simulink model "hybrid_lht_accumulator_backup"  (R2019b)
settings: Solver=FixedStepDiscrete  StartTime=0.0  StopTime=inf  FixedStep=1/bt.frequency  RelTol=1e-3
InitFcn:
  | ht_hybrid_setup;
StopFcn:
  | ht_hybrid_compare;
undefined symbols (not defined in the file or in its folder): bt, height, Ntheta, nTheta, width
libraries: hdlsllib x52, simulink x24, visionhdlutilities x2, dspsrcs4 x1, visionhdlio x1, lib_hybrid_ht_kernel x1, visionsources x1
(part 4 of 5)

== system hybrid_lht_accumulator_backup/Hybrid LHT2/Hybrid LHT Accumulator/Accumulator with Switches/Accumulator/Block RAM ==
  wr_data : Inport
  wr_addr : Inport  Port=2
  wr_en : Inport  Port=3
  rd_addr : Inport  Port=4
  Simple Dual Port RAM : Subsystem  VariantControl=9_bits
  Simple Dual Port RAM Generator : Subsystem  VariantControl=other_bits  mask{b=36, d=400, b_hidden=12, d_hidden=2204}
      mask prompts: b "Data width:"; d "Depth:"
      mask init:
      | if b == b_hidden && d == d_hidden
      |     return
      | end
      | 
      | % Xilinx RAM Initialisation
      | xl_config = [512, 72;
      |             1024, 36;
      |             2048, 18;
      |             4096, 9;
      |             8192, 4;
      |             16384, 2;
      |             32768, 1];
      | 
      | % Get length of Xilinx Configuration
      | sizeram = size(xl_config);
      |         
      | % Get the RAM Configuration based on the data width
      | for i = 1:sizeram(1)
      |     if b <= xl_config(i, 2)
      |         a = xl_config(i, :);
      |     end
      | end
      | 
      | % Get number of BRAM required (including half BRAM)
      | numbram = ceil((d/a(1))/0.5)*0.5;
      | fullbram = floor(numbram); % Integer
      | halfbram = (numbram-floor(numbram)) ~= 0; % Boolean
      | 
      | % Get all blocks and delete everything excepts ports
      | H = get(find_system(gcb, 'FindAll', 'on', 'type', 'block'));
      | todelete = setdiff(strcat(repmat({[gcb '/']}, numel(H.Blocks), 1),  H.Blocks),...
      |     strcat(repmat({[gcb '/']}, 5, 1),...
      |     {'wr_data'; 'wr_addr'; 'wr_en'; 'rd_addr'; 'rd_data'}));
      | delete_block(todelete);
      | 
      | % Delete lines
      | for i = 1:numel(H.Lines)
      |     delete_line(H.Lines(i).Handle)
      | end
      | 
      | % Generate full BRAMs
      | y = 0;
      | 
      | % If there is only one ram then the write enable should be directly
      | % connected to the first ram write enable. Else, the write address must be sliced
      | % and the upper bound (over a(2)) compared to zero. This will indicate if
      | % the first ram is the one to be written/read from.
      | 
      | % Common to both implementations
      | % Write Address Slice
      | add_block('hdlsllib/Logic and Bit Operations/Bit Slice',...
      |         [gcb, '/wr_address'], 'Position',...
      |         [160 130 250 170]);
      | % Set bitslice parameters
      | set_param([gcb, '/wr_address'],...
      |     'lidx', int2str(log2(a(1))-1));
      | set_param([gcb, '/wr_address'],...
      |     'ridx', int2str(0));
      | 
      | % Read Address Slice
      | add_block('hdlsllib/Logic and Bit Operations/Bit Slice',...
      |         [gcb, '/rd_address'], 'Position',...
      |         [160 330 250 370]);
      | % Set bitslice parameters
      | set_param([gcb, '/rd_address'],...
      |     'lidx', int2str(log2(a(1))-1));
      | set_param([gcb, '/rd_address'],...
      |     'ridx', int2str(0));
      | 
      | if ceil(numbram) == 1
      |     
      |     i = 1;
      |     
      |     % Add Simple RAM
      |     add_block('hdlsllib/HDL RAMs/Simple Dual Port RAM',...
      |         [gcb, '/simple_ram_', int2str(i-1)], 'Position',...
      |         [635 0+600*y 635+200 400+600*y]);
      | 
      |     % Set RAM parameters
      |     set_param([gcb, '/simple_ram_', int2str(i-1)],...
      |         'ram_size', int2str(log2(a(1))));
      | 
      |     % Connect "wr_data" to "simple_ram_i"
      |     add_line(gcb, ['wr_data/1'], ['simple_ram_', int2str(i-1), '/1'],...
      |         'autorouting', 'on');
      |     
      |     % Connect "wr_addr" to "wr_address"
      |     add_line(gcb, ['wr_addr/1'], ['wr_address/1'],...
      |         'autorouting', 'on');
      | 
      |     % Connect "wr_address" to "simple_ram_i"
      |     add_line(gcb, ['wr_address/1'], ['simple_ram_', int2str(i-1), '/2'],...
      |         'autorouting', 'on');
      | 
      |     % Connect "wr_en" to "simple_ram_i"
      |     add_line(gcb, ['wr_en/1'], ['simple_ram_', int2str(i-1), '/3'],...
      |         'autorouting', 'on');
      |     
      |     % Connect "rd_addr" to "rd_address"
      |     add_line(gcb, ['rd_addr/1'], ['rd_address/1'],...
      |         'autorouting', 'on');
      | 
      |     % Connect "rd_address" to "simple_ram_i"
      |     add_line(gcb, ['rd_address/1'], ['simple_ram_', int2str(i-1), '/4'],...
      |         'autorouting', 'on');
      | 
      |     % Connect "simple_ram_i" to "rd_data"
      |     add_line(gcb, ['simple_ram_', int2str(i-1), '/1'], ['rd_data/1'],...
      |         'autorouting', 'on');
      | 
      | else
      |     
      |     % Multiport Switch
      |     add_block('hdlsllib/Signal Routing/Multiport Switch',...
      |         [gcb, '/multiport_switch'], 'Position',...
      |         [1340 146 1405 250]);
      |     % Set multiport switch parameters
      |     set_param([gcb, '/multiport_switch'],...
      |         'Inputs', int2str(ceil(numbram)));
      |     set_param([gcb, '/multiport_switch'],...
      |         'DataPortOrder', 'Zero-based contiguous');
      | 
      |     % Add Constant Zero
      |     add_block('hdlsllib/Sources/Constant',...
      |         [gcb, '/zero'], 'Position',...
      |         [425 -65 455 -35]);
      |     set_param([gcb, '/zero'],...
      |         'Value', int2str(0));
      |     set_param([gcb, '/zero'],...
      |         'OutDataTypeStr', ['fixdt(0, ', int2str(ceil(numbram)), ', 0)']);
      | 
      |     % Add Vector Concatenate
      |     add_block('hdlsllib/Signal Routing/Vector Concatenate',...
      |         [gcb, '/vector_concatenate'], 'Position',...
      |         [1015, -113, 1025, 38]);
      |     set_param([gcb, '/vector_concatenate'],...
      |         'NumInputs', int2str(ceil(numbram)));
      | 
      |     % Add Bitwise-OR
      |     add_block('hdlsllib/Logic and Bit Operations/Bitwise Operator',...
      |         [gcb, '/bitwise_or'], 'Position',...
      |         [1165, -54, 1205, -16]);
      |     set_param([gcb, '/bitwise_or'],...
      |         'logicop', 'OR');
      |     set_param([gcb, '/bitwise_or'],...
      |         'UseBitMask', 0);
      |     set_param([gcb, '/bitwise_or'],...
      |         'NumInputPorts', int2str(1));
      | 
      |     % Add delay for bram access
      |     add_block('hdlsllib/Discrete/Delay',...
      |         [gcb, '/delay'], 'Position',...
      |         [1248, 60, 1282, 95]);
      |     set_param([gcb, '/delay'],...
      |         'DelayLength', int2str(1));
      |     
      |     % Add bitslice
      |     add_block('hdlsllib/Logic and Bit Operations/Bit Slice',...
      |         [gcb, '/wr_bitslice'], 'Position',...
      |         [-65 180 25 220]);
      | 
      |     % Set bitslice parameters
      |     set_param([gcb, '/wr_bitslice'],...
      |         'lidx', int2str(ceil(log2(d)-1)));
      |     set_param([gcb, '/wr_bitslice'],...
      |         'ridx', int2str(log2(a(1))));
      |     
      |     % Add bitslice
      |     add_block('hdlsllib/Logic and Bit Operations/Bit Slice',...
      |         [gcb, '/rd_bitslice'], 'Position',...
      |         [-65 280 25 320]);
      | 
      |     % Set bitslice parameters
      |     set_param([gcb, '/rd_bitslice'],...
      |         'lidx', int2str(ceil(log2(d)-1)));
      |     set_param([gcb, '/rd_bitslice'],...
      |         'ridx', int2str(log2(a(1))));
      |     
      |     for i = 1:ceil(numbram)
      |         
      |         %%%%% Begin Adding Blocks %%%%%
      |         % Add Simple RAM
      |         add_block('hdlsllib/HDL RAMs/Simple Dual Port RAM',...
      |             [gcb, '/simple_ram_', int2str(i-1)], 'Position',...
      |             [635 0+600*y 635+200 400+600*y]);
      | 
      |         % Set RAM parameters
      |         set_param([gcb, '/simple_ram_', int2str(i-1)],...
      |             'ram_size', int2str(log2(a(1))));
      | 
      |         % Add compare to constant
      |         add_block('hdlsllib/Logic and Bit Operations/Compare To Constant',...
      |             [gcb, '/wr_cmp2const_', int2str(i-1)], 'Position',...
      |             [190 225+y*600 220 255+y*600]); 
      | 
      |         % Set compare to zero parameters
      |         set_param([gcb, '/wr_cmp2const_', int2str(i-1)],...
      |             'relop', '==');
      | 
      |         % Set compare to zero parameters
      |         set_param([gcb, '/wr_cmp2const_', int2str(i-1)],...
      |             'const', int2str(i-1));
      |         
      |         % Add compare to constant
      |         add_block('hdlsllib/Logic and Bit Operations/Compare To Constant',...
      |             [gcb, '/rd_cmp2const_', int2str(i-1)], 'Position',...
      |             [190 445+y*600 220 475+y*600]); 
      | 
      |         % Set compare to zero parameters
      |         set_param([gcb, '/rd_cmp2const_', int2str(i-1)],...
      |             'relop', '==');
      | 
      |         % Set compare to zero parameters
      |         set_param([gcb, '/rd_cmp2const_', int2str(i-1)],...
      |             'const', int2str(i-1));
      | 
      |         % Add and logic
      |         add_block('hdlsllib/Logic and Bit Operations/Logical Operator',...
      |             [gcb, '/and_', int2str(i-1)], 'Position',...
      |             [420 231+600*y 455 264+600*y]);
      | 
      |         % Set and logic parameters
      |         set_param([gcb, '/and_', int2str(i-1)],...
      |             'Operator', 'AND');
      | 
      |         % Add Switch
      |         add_block('hdlsllib/Signal Routing/Switch',...
      |             [gcb, '/switch_', int2str(i-1)], 'Position',...
      |             [685 -113+600*y 785 -37+600*y]);
      | 
      |         % Set switch parameters
      |         set_param([gcb, '/switch_', int2str(i-1)],...
      |             'Threshold', int2str(1));
      | 
      |         % Add Constant
      |         add_block('hdlsllib/Sources/Constant',...
      |             [gcb, '/constant_', int2str(i-1)], 'Position',...
      |             [425 -115+600*y 455 -85+600*y]);
      | 
      |         % Set Constant parameters
      |         set_param([gcb, '/constant_', int2str(i-1)],...
      |             'Value', int2str(i-1));
      |         set_param([gcb, '/constant_', int2str(i-1)],...
      |             'OutDataTypeStr', ['fixdt(0, ', int2str(ceil(numbram)), ', 0)']);   
      | 
      |         %%%%% Begin Wire Connections %%%%%        
      |         % Connect "wr_data" to "simple_ram_i"
      |         add_line(gcb, 'wr_data/1', ['simple_ram_', int2str(i-1), '/1'],...
      |             'autorouting','on');
      | 
      |         % Connect "wr_address" to "simple_ram_i"
      |         add_line(gcb, 'wr_address/1', ['simple_ram_', int2str(i-1), '/2'],...
      |             'autorouting','on');
      | 
      |         % Connect "rd_address" to "simple_ram_i"
      |         add_line(gcb, 'rd_address/1', ['simple_ram_', int2str(i-1), '/4'],...
      |             'autorouting','on');
      | 
      |         % Connect "constant_i" to "switch_i"
      |         add_line(gcb, ['constant_', int2str(i-1), '/1'], ['switch_', int2str(i-1), '/1'],...
      |             'autorouting','on');
      | 
      |         % Connect "zero" to "switch_i"
      |         add_line(gcb, 'zero/1', ['switch_', int2str(i-1), '/3'],...
      |             'autorouting','on');
      | 
      |         % Connect "switch_i" to "vector_concatenate"
      |         add_line(gcb, ['switch_', int2str(i-1), '/1'], ['vector_concatenate/', int2str(i)],...
      |             'autorouting','on');
      | 
      |         % Connect "rd_address" to "simple_ram_i"
      |         add_line(gcb, ['simple_ram_', int2str(i-1), '/1'],['multiport_switch/', int2str(i+1)],...
      |             'autorouting','on');
      | 
      |         % Connect "bitslice_i" to "wr_cmp2const_i"
      |         add_line(gcb, ['wr_bitslice/1'], ['wr_cmp2const_', int2str(i-1), '/1'],...
      |             'autorouting','on');
      |         
      |         % Connect "bitslice_i" to "rd_cmp2const_i"
      |         add_line(gcb, ['rd_bitslice/1'], ['rd_cmp2const_', int2str(i-1), '/1'],...
      |             'autorouting','on');
      | 
      |         % Connect "wr_en" to "and_i"
      |         add_line(gcb, ['wr_en/1'], ['and_', int2str(i-1), '/2'],...
      |             'autorouting','on');
      | 
      |         % Connect "and_i" to "simple_ram_0"
      |         add_line(gcb, ['and_', int2str(i-1), '/1'], ['simple_ram_', int2str(i-1), '/3'],...
      |             'autorouting','on');
      | 
      |         % Connect "wr_cmp2const_i" to "and_i"
      |         add_line(gcb, ['wr_cmp2const_', int2str(i-1), '/1'], ['and_', int2str(i-1), '/1'],...
      |             'autorouting','on');
      | 
      |         % Connect "rd_cmp2const_i" to "switch_i"
      |         add_line(gcb, ['rd_cmp2const_', int2str(i-1), '/1'], ['switch_', int2str(i-1), '/2'],...
      |             'autorouting','on');
      |          
      |         % Update coordinates
      |         y = y + 1;
      |         
      |     end
      |     
      |     % Connect "rd_addr" to "bitslice_i"
      |     add_line(gcb, ['rd_addr/1'], ['rd_bitslice/1'],...
      |         'autorouting','on');
      |     
      |     % Connect "wr_addr" to "bitslice_i"
      |     add_line(gcb, ['wr_addr/1'], ['wr_bitslice/1'],...
      |         'autorouting','on');
      |     
      |     % Connect "wr_addr" to "wr_address"
      |     add_line(gcb, 'wr_addr/1', ['wr_address', '/1'],...
      |         'autorouting','on');
      | 
      |     % Connect "rd_addr" to "rd_address"
      |     add_line(gcb, 'rd_addr/1', ['rd_address', '/1'],...
      |         'autorouting','on');
      | 
      |     % Connect "vector_concatenate" to "bitwise_or"
      |     add_line(gcb, ['vector_concatenate/1'], ['bitwise_or/1'],...
      |         'autorouting','on');
      | 
      |     % Connect "bitwise_or" to "delay"
      |     add_line(gcb, ['bitwise_or/1'], ['delay/1'],...
      |         'autorouting','on');
      | 
      |     % Connect "delay" to "multiport_switch"
      |     add_line(gcb, ['delay/1'], ['multiport_switch/1'],...
      |         'autorouting','on');
      | 
      |     % Connect "multiport_switch" to "rd_data"
      |     add_line(gcb, ['multiport_switch/1'], ['rd_data/1'],...
      |         'autorouting','on');
      |     
      | end
      | 
      | % If there is a half bram we must change a few parameters. Firstly, delete
      | % the write and read address lines. Then add bitslice blocks to reduce the
      | % address space in half. Connect rd_addr and wr_addr to the corresponding ports
      | % on the bram. Finally, change the address depth.
      | if halfbram
      |     
      |     if ceil(numbram) > 1
      |         
      |         % Delete lines
      |         delete_line(gcb, ['wr_address/1'], ['simple_ram_', int2str(i-1), '/2'])
      |         delete_line(gcb, ['rd_address/1'], ['simple_ram_', int2str(i-1), '/4'])
      |         
      |         % Write Address half ram Slice
      |         add_block('hdlsllib/Logic and Bit Operations/Bit Slice',...
      |                 [gcb, '/wr_address_hr'], 'Position',...
      |                 [160 130+(y-1)*600 250 170+(y-1)*600]);
      |         % Set bitslice parameters
      |         set_param([gcb, '/wr_address_hr'],...
      |             'lidx', int2str(log2(a(1))-2));
      |         set_param([gcb, '/wr_address_hr'],...
      |             'ridx', int2str(0));
      | 
      |         % Read Address half ram Slice
      |         add_block('hdlsllib/Logic and Bit Operations/Bit Slice',...
      |                 [gcb, '/rd_address_hr'], 'Position',...
      |                 [160 330+(y-1)*600 250 370+(y-1)*600]);
      |         % Set bitslice parameters
      |         set_param([gcb, '/rd_address_hr'],...
      |             'lidx', int2str(log2(a(1))-2));
      |         set_param([gcb, '/rd_address_hr'],...
      |             'ridx', int2str(0));
      | 
      |         % Connect "wr_addr" to "wr_address_hr"
      |         add_line(gcb, 'wr_addr/1', ['wr_address_hr', '/1'],...
      |             'autorouting','on');
      | 
      |         % Connect "rd_addr" to "rd_address_hr"
      |         add_line(gcb, 'rd_addr/1', ['rd_address_hr', '/1'],...
      |             'autorouting','on');
      | 
      |         % Connect "wr_address_hr" to "simple_ram_i"
      |         add_line(gcb, ['wr_address_hr', '/1'], ['simple_ram_', int2str(i-1), '/2'],...
      |             'autorouting','on');
      | 
      |         % Connect "rd_address_hr" to "simple_ram_i"
      |         add_line(gcb, ['rd_address_hr', '/1'], ['simple_ram_', int2str(i-1), '/4'],...
      |             'autorouting','on');
      | 
      |     else
      |         % Set bitslice parameters
      |         set_param([gcb, '/wr_address'],...
      |             'lidx', int2str(log2(a(1))-2));
      |         set_param([gcb, '/wr_address'],...
      |             'ridx', int2str(0));
      |         % Set bitslice parameters
      |         set_param([gcb, '/rd_address'],...
      |             'lidx', int2str(log2(a(1))-2));
      |         set_param([gcb, '/rd_address'],...
      |             'ridx', int2str(0));
      |         
      |     end
      |     
      |     % Update the ram parameters (address bits)
      |     set_param([gcb, '/simple_ram_', int2str(i-1)],...
      |         'ram_size', int2str(log2(a(1)/2)));
      |     
      | end
      | 
      | b_hidden = b;
      | d_hiddne = d;
  rd_data : Outport

== system hybrid_lht_accumulator_backup/Hybrid LHT2/Hybrid LHT Accumulator2/Simple Hough Accumulator/Flag Generator/Flag Generator ==
  ReadOut : Inport
  Thresh : Inport  Port=2
  ZeroData : Inport  Port=3
  ReadValid : Inport  Port=4
  AND : Logic  IconShape=distinctive  AllPortsSameDT=off  OutDataTypeStr=boolean
  Bit Concat : hdlsllib/Logic and Bit Operations/Bit Concat  numInputs=2
      settings: SourceProductName=HDL Coder  SourceProductBaseCode=HD
  Relational Operator1 : RelationalOperator  OutDataTypeStr=boolean  RndMeth=Simplest
  ZeroDataFlagged : Outport  VectorParamsAs1DForOutWhenUnconnected=off
  wires:
  AND/1 -> Bit Concat/1
  ReadValid/1 -> AND/2
  Relational Operator1/1 -> AND/1
  ZeroData/1 -> Bit Concat/2
  Bit Concat/1 -> ZeroDataFlagged/1
  Thresh/1 -> Relational Operator1/2
  ReadOut/1 -> Relational Operator1/1

== system hybrid_lht_accumulator_backup/Hybrid LHT2/Hybrid LHT Accumulator2/Simple Hough Accumulator/Flag Generator/Passthrough ==
  ZeroData : Inport
  ZeroDataFlagged : Outport  VectorParamsAs1DForOutWhenUnconnected=off
  wires:
  ZeroData/1 -> ZeroDataFlagged/1

== system hybrid_lht_accumulator_backup/Hybrid LHT2/Hybrid LHT Accumulator2/Simple Hough Accumulator/Hough Accumulator/Simple Dual Port RAM Generator ==
  wr_data : Inport
  wr_addr : Inport  Port=2
  wr_en : Inport  Port=3
  rd_addr : Inport  Port=4
  rd_address : hdlsllib/Logic and Bit Operations/Bit Slice  lidx=8  ridx=0
      settings: SourceProductName=Simulink  SourceProductBaseCode=SL
  simple_ram_0 : hdlsllib/HDL RAMs/Simple Dual Port RAM  ram_size=9
      settings: SourceProductName=Simulink  SourceProductBaseCode=SL
  wr_address : hdlsllib/Logic and Bit Operations/Bit Slice  lidx=8  ridx=0
      settings: SourceProductName=Simulink  SourceProductBaseCode=SL
  rd_data : Outport
  wires:
  wr_data/1 -> simple_ram_0/1
  wr_addr/1 -> wr_address/1
  wr_address/1 -> simple_ram_0/2
  wr_en/1 -> simple_ram_0/3
  rd_addr/1 -> rd_address/1
  rd_address/1 -> simple_ram_0/4
  simple_ram_0/1 -> rd_data/1

== system hybrid_lht_accumulator_backup/Hybrid LHT2/Hybrid LHT Accumulator2/Simple Hough Accumulator/Keep Flag/Keep Flag ==
  FlagIn : Inport
  VoteIn : Inport  Port=2
  Bit Concat1 : hdlsllib/Logic and Bit Operations/Bit Concat  numInputs=2
      settings: SourceProductName=HDL Coder  SourceProductBaseCode=HD
  VoteFlagOut : Outport  VectorParamsAs1DForOutWhenUnconnected=off
  wires:
  VoteIn/1 -> Bit Concat1/2
  FlagIn/1 -> Bit Concat1/1
  Bit Concat1/1 -> VoteFlagOut/1

== system hybrid_lht_accumulator_backup/Hybrid LHT2/Hybrid LHT Accumulator2/Simple Hough Accumulator/Keep Flag/Passthrough ==
  FlagIn : Inport
  VoteIn : Inport  Port=2
  Terminator : Terminator
  VoteFlagOut : Outport  VectorParamsAs1DForOutWhenUnconnected=off
  wires:
  VoteIn/1 -> VoteFlagOut/1
  FlagIn/1 -> Terminator/1

== system hybrid_lht_accumulator_backup/Hybrid LHT2/Hybrid LHT Accumulator2/Simple Hough Accumulator/Separate Bits/Passthrough ==
  VoteFlagIn : Inport
  Constant : Constant  Value=0  OutDataTypeStr=boolean  SampleTime=-1
  FlagOut : Outport  VectorParamsAs1DForOutWhenUnconnected=off
  VoteOut : Outport  Port=2  VectorParamsAs1DForOutWhenUnconnected=off
  wires:
  VoteFlagIn/1 -> VoteOut/1
  Constant/1 -> FlagOut/1

== system hybrid_lht_accumulator_backup/Hybrid LHT2/Hybrid LHT Accumulator2/Simple Hough Accumulator/Separate Bits/Separate Bits ==
  VoteFlagIn : Inport
  Bit Slice : hdlsllib/Logic and Bit Operations/Bit Slice  lidx=voteWL-2  ridx=0
  Bit Slice1 : hdlsllib/Logic and Bit Operations/Bit Slice  lidx=voteWL-1  ridx=voteWL-1
  FlagOut : Outport  VectorParamsAs1DForOutWhenUnconnected=off
  VoteOut : Outport  Port=2  VectorParamsAs1DForOutWhenUnconnected=off
  wires:
  VoteFlagIn/1 -> Bit Slice/1, Bit Slice1/1
  Bit Slice/1 -> VoteOut/1
  Bit Slice1/1 -> FlagOut/1

== system hybrid_lht_accumulator_backup/Hybrid LHT2/Hybrid LHT Kernel/Gradient Kernel System/Get Index and Fix Limits/Extract Active Votes ==
  note: Check the indices to ensure they are in the correct limits
  Theta : Inport
  Add : Sum
  Add1 : Sum  Inputs=+-
  Add3 : Sum
  Constant : Constant  Value=[-lambda:1:lambda-subflag]  VectorParams1D=off  OutDataTypeStr=fixdt(1,ceil(log2(lambda+1))+1, 0)  SampleTime=-1
  Data Type Conversion : DataTypeConversion  OutDataTypeStr=fixdt(0, ceil(log2(nTheta+1)), 0)
  High : Constant  Value=nTheta-1  OutDataTypeStr=fixdt(0,ceil(log2(nTheta)),0)  SampleTime=-1
  Low : Constant  Value=0  OutDataTypeStr=fixdt(0,1,0)  SampleTime=-1
  Multiport Switch2 : MultiPortSwitch  DataPortOrder=Zero-based contiguous  Inputs=2  zeroidx=on
  Multiport Switch3 : MultiPortSwitch  DataPortOrder=Zero-based contiguous  Inputs=2  zeroidx=on
  Relational : RelationalOperator  Operator=<  OutDataTypeStr=boolean  RndMeth=Nearest
  Relational1 : RelationalOperator  Operator=>  OutDataTypeStr=boolean  RndMeth=Nearest
  nTheta : Constant  Value=nTheta  OutDataTypeStr=fixdt(0,ceil(log2(nTheta+1)),0)  SampleTime=-1
  Index : Outport  VectorParamsAs1DForOutWhenUnconnected=off
  wires:
  Data Type Conversion/1 -> Index/1
  Theta/1 -> Add/1
  Add/1 -> Multiport Switch2/2, Relational/1, Add3/1
  nTheta/1 -> Add1/2, Add3/2
  Multiport Switch2/1 -> Multiport Switch3/2, Relational1/1, Add1/1
  Low/1 -> Relational/2
  Add3/1 -> Multiport Switch2/3
  Relational1/1 -> Multiport Switch3/1
  High/1 -> Relational1/2
  Multiport Switch3/1 -> Data Type Conversion/1
  Relational/1 -> Multiport Switch2/1
  Add1/1 -> Multiport Switch3/3
  Constant/1 -> Add/2

== system hybrid_lht_accumulator_backup/Hybrid LHT2/Hybrid LHT Kernel/Gradient Kernel System/Get Index and Fix Limits/GetShift1 ==
  Theta : Inport  Partition=on  PartitionDimension=2  PartitionWidth=1  PartitionOffset=0
  Add : Sum  Inputs=+  OutDataTypeStr=fixdt(0, ceil(log2(L+1)), 0)
  Constant : Constant  Value=U  VectorParams1D=off  OutDataTypeStr=fixdt(0,ceil(log2(max(U)+1)),0)  SampleTime=-1
  For Each : ForEach  DisableCoverage=on
  Relational Operator : RelationalOperator  OutDataTypeStr=boolean  RndMeth=Nearest
  Shift : Outport  ConcatenationDimension=2  VectorParamsAs1DForOutWhenUnconnected=off
  wires:
  Relational Operator/1 -> Add/1
  Add/1 -> Shift/1
  Theta/1 -> Relational Operator/1
  Constant/1 -> Relational Operator/2

== system hybrid_lht_accumulator_backup/Hybrid LHT2/Hybrid LHT Kernel/Gradient Kernel System/Hough Kernel/Hough Kernel ==
  X : Inport
  Y : Inport  Port=2
  Index : Inport  Port=3
  Add : Sum  OutDataTypeStr=fixdt(1, ceil(log2(2*maxRho)), 0)  RndMeth=Round
  CosineROM : Constant  Value=fi(cos(deg2rad(theta)), 1, 16, 14)  VectorParams1D=off  OutDataTypeStr=fixdt(1,16,14)  SampleTime=-1
  Selector : Selector  NumberOfDimensions=2  IndexMode=Zero-based  InputPortWidth=3  IndexOptions=Index vector (dialog),Index vector (port)  Indices=0,1  OutputSizes=1,1
  Selector1 : Selector  NumberOfDimensions=2  IndexMode=Zero-based  InputPortWidth=3  IndexOptions=Index vector (dialog),Index vector (port)  Indices=0,1  OutputSizes=1,1
  SineROM : Constant  Value=fi(sin(deg2rad(theta)), 1, 16, 14)  VectorParams1D=off  OutDataTypeStr=fixdt(1,16,14)  SampleTime=-1
  xcos : Product  OutDataTypeStr=fixdt(1, ceil(log2(width+1)), 0);  RndMeth=Round
  ysin : Product  OutDataTypeStr=fixdt(1, ceil(log2(height+1)), 0);  RndMeth=Round
  Rho : Outport  VectorParamsAs1DForOutWhenUnconnected=off
  wires:
  CosineROM/1 -> Selector/1
  Selector/1 -> xcos/2
  xcos/1 -> Add/1
  Y/1 -> ysin/1
  Add/1 -> Rho/1
  SineROM/1 -> Selector1/1
  ysin/1 -> Add/2
  Selector1/1 -> ysin/2
  X/1 -> xcos/1
  Index/1 -> Selector/2, Selector1/2

== system hybrid_lht_accumulator_backup/Hybrid LHT2/Hybrid LHT Kernel1/Gradient Kernel System/Extract Active Votes/GetShift ==
  Theta : Inport
  Add : Sum  Inputs=+  OutDataTypeStr=fixdt(0, ceil(log2(L+1)), 0)
  Constant : Constant  Value=U  VectorParams1D=off  OutDataTypeStr=fixdt(0,ceil(log2(max(U)+1)),0)  SampleTime=-1
  Relational Operator : RelationalOperator  OutDataTypeStr=boolean  RndMeth=Nearest
  Shift : Outport  VectorParamsAs1DForOutWhenUnconnected=off
  wires:
  Constant/1 -> Relational Operator/2
  Theta/1 -> Relational Operator/1
  Add/1 -> Shift/1
  Relational Operator/1 -> Add/1

== system hybrid_lht_accumulator_backup/Hybrid LHT2/Hybrid LHT Kernel1/Gradient Kernel System/Get Index and Fix Limits/Extract Active Votes ==
  note: Check the indices to ensure they are in the correct limits
  Theta : Inport
  Add : Sum
  Add1 : Sum  Inputs=+-
  Add3 : Sum
  Constant : Constant  Value=[-lambda:1:lambda-subflag]  VectorParams1D=off  OutDataTypeStr=fixdt(1,ceil(log2(lambda+1))+1, 0)  SampleTime=-1
  Data Type Conversion : DataTypeConversion  OutDataTypeStr=fixdt(0, ceil(log2(nTheta+1)), 0)
  High : Constant  Value=nTheta-1  OutDataTypeStr=fixdt(0,ceil(log2(nTheta)),0)  SampleTime=-1
  Low : Constant  Value=0  OutDataTypeStr=fixdt(0,1,0)  SampleTime=-1
  Multiport Switch2 : MultiPortSwitch  DataPortOrder=Zero-based contiguous  Inputs=2  zeroidx=on
  Multiport Switch3 : MultiPortSwitch  DataPortOrder=Zero-based contiguous  Inputs=2  zeroidx=on
  Relational : RelationalOperator  Operator=<  OutDataTypeStr=boolean  RndMeth=Nearest
  Relational1 : RelationalOperator  Operator=>  OutDataTypeStr=boolean  RndMeth=Nearest
  nTheta : Constant  Value=nTheta  OutDataTypeStr=fixdt(0,ceil(log2(nTheta+1)),0)  SampleTime=-1
  Index : Outport  VectorParamsAs1DForOutWhenUnconnected=off
  wires:
  Constant/1 -> Add/2
  Add1/1 -> Multiport Switch3/3
  Relational/1 -> Multiport Switch2/1
  Multiport Switch3/1 -> Data Type Conversion/1
  High/1 -> Relational1/2
  Relational1/1 -> Multiport Switch3/1
  Add3/1 -> Multiport Switch2/3
  Low/1 -> Relational/2
  Multiport Switch2/1 -> Add1/1, Relational1/1, Multiport Switch3/2
  nTheta/1 -> Add3/2, Add1/2
  Add/1 -> Add3/1, Relational/1, Multiport Switch2/2
  Theta/1 -> Add/1
  Data Type Conversion/1 -> Index/1

== system hybrid_lht_accumulator_backup/Hybrid LHT2/Hybrid LHT Kernel1/Gradient Kernel System/Get Index and Fix Limits/GetShift1 ==
  Theta : Inport  Partition=on  PartitionDimension=2  PartitionWidth=1  PartitionOffset=0
  Add : Sum  Inputs=+  OutDataTypeStr=fixdt(0, ceil(log2(L+1)), 0)
  Constant : Constant  Value=U  VectorParams1D=off  OutDataTypeStr=fixdt(0,ceil(log2(max(U)+1)),0)  SampleTime=-1
  For Each : ForEach  DisableCoverage=on
  Relational Operator : RelationalOperator  OutDataTypeStr=boolean  RndMeth=Nearest
  Shift : Outport  ConcatenationDimension=2  VectorParamsAs1DForOutWhenUnconnected=off
  wires:
  Constant/1 -> Relational Operator/2
  Theta/1 -> Relational Operator/1
  Add/1 -> Shift/1
  Relational Operator/1 -> Add/1

== system hybrid_lht_accumulator_backup/Hybrid LHT2/Hybrid LHT Kernel1/Gradient Kernel System/Hough Kernel/Hough Kernel ==
  X : Inport
  Y : Inport  Port=2
  Index : Inport  Port=3
  Add : Sum  OutDataTypeStr=fixdt(1, ceil(log2(2*maxRho)), 0)  RndMeth=Round
  CosineROM : Constant  Value=fi(cos(deg2rad(theta)), 1, 16, 14)  VectorParams1D=off  OutDataTypeStr=fixdt(1,16,14)  SampleTime=-1
  Selector : Selector  NumberOfDimensions=2  IndexMode=Zero-based  InputPortWidth=3  IndexOptions=Index vector (dialog),Index vector (port)  Indices=0,1  OutputSizes=1,1
  Selector1 : Selector  NumberOfDimensions=2  IndexMode=Zero-based  InputPortWidth=3  IndexOptions=Index vector (dialog),Index vector (port)  Indices=0,1  OutputSizes=1,1
  SineROM : Constant  Value=fi(sin(deg2rad(theta)), 1, 16, 14)  VectorParams1D=off  OutDataTypeStr=fixdt(1,16,14)  SampleTime=-1
  xcos : Product  OutDataTypeStr=fixdt(1, ceil(log2(width+1)), 0);  RndMeth=Round
  ysin : Product  OutDataTypeStr=fixdt(1, ceil(log2(height+1)), 0);  RndMeth=Round
  Rho : Outport  VectorParamsAs1DForOutWhenUnconnected=off
  wires:
  Index/1 -> Selector1/2, Selector/2
  X/1 -> xcos/1
  Selector1/1 -> ysin/2
  ysin/1 -> Add/2
  SineROM/1 -> Selector1/1
  Add/1 -> Rho/1
  Y/1 -> ysin/1
  xcos/1 -> Add/1
  Selector/1 -> xcos/2
  CosineROM/1 -> Selector/1

== system hybrid_lht_accumulator_backup/Hybrid LHT2/Hybrid LHT Kernel2/Gradient Kernel System/Get Index and Fix Limits/Extract Active Votes ==
  note: Check the indices to ensure they are in the correct limits
  Theta : Inport
  Add : Sum
  Add1 : Sum  Inputs=+-
  Add3 : Sum
  Constant : Constant  Value=[-lambda:1:lambda-subflag]  VectorParams1D=off  OutDataTypeStr=fixdt(1,ceil(log2(lambda+1))+1, 0)  SampleTime=-1
  Data Type Conversion : DataTypeConversion  OutDataTypeStr=fixdt(0, ceil(log2(Ntheta+1)), 0)
  High : Constant  Value=Ntheta-1  OutDataTypeStr=fixdt(0,ceil(log2(Ntheta)),0)  SampleTime=-1
  Low : Constant  Value=0  OutDataTypeStr=fixdt(0,1,0)  SampleTime=-1
  Multiport Switch2 : MultiPortSwitch  DataPortOrder=Zero-based contiguous  Inputs=2  zeroidx=on
  Multiport Switch3 : MultiPortSwitch  DataPortOrder=Zero-based contiguous  Inputs=2  zeroidx=on
  Relational : RelationalOperator  Operator=<  OutDataTypeStr=boolean  RndMeth=Nearest
  Relational1 : RelationalOperator  Operator=>  OutDataTypeStr=boolean  RndMeth=Nearest
  nTheta : Constant  Value=Ntheta  OutDataTypeStr=fixdt(0,ceil(log2(Ntheta+1)),0)  SampleTime=-1
  Index : Outport  VectorParamsAs1DForOutWhenUnconnected=off
  wires:
  Constant/1 -> Add/2
  Add1/1 -> Multiport Switch3/3
  Relational/1 -> Multiport Switch2/1
  Multiport Switch3/1 -> Data Type Conversion/1
  High/1 -> Relational1/2
  Relational1/1 -> Multiport Switch3/1
  Add3/1 -> Multiport Switch2/3
  Low/1 -> Relational/2
  Multiport Switch2/1 -> Add1/1, Relational1/1, Multiport Switch3/2
  nTheta/1 -> Add3/2, Add1/2
  Add/1 -> Add3/1, Relational/1, Multiport Switch2/2
  Theta/1 -> Add/1
  Data Type Conversion/1 -> Index/1

== system hybrid_lht_accumulator_backup/Hybrid LHT2/Hybrid LHT Kernel2/Gradient Kernel System/Get Index and Fix Limits/GetShift1 ==
  Theta : Inport  Partition=on  PartitionDimension=2  PartitionWidth=1  PartitionOffset=0
  Add : Sum  Inputs=+  OutDataTypeStr=fixdt(0, ceil(log2(L+1)), 0)
  Constant : Constant  Value=U  VectorParams1D=off  OutDataTypeStr=fixdt(0,ceil(log2(max(U)+1)),0)  SampleTime=-1
  For Each : ForEach  DisableCoverage=on
  Relational Operator : RelationalOperator  OutDataTypeStr=boolean  RndMeth=Nearest
  Shift : Outport  ConcatenationDimension=2  VectorParamsAs1DForOutWhenUnconnected=off
  wires:
  Constant/1 -> Relational Operator/2
  Theta/1 -> Relational Operator/1
  Add/1 -> Shift/1
  Relational Operator/1 -> Add/1

== system hybrid_lht_accumulator_backup/Hybrid LHT2/Hybrid LHT Kernel2/Gradient Kernel System/Hough Kernel/Hough Kernel ==
  X : Inport
  Y : Inport  Port=2
  Index : Inport  Port=3
  Add : Sum  OutDataTypeStr=fixdt(1, ceil(log2(2*maxRho)), 0)  RndMeth=Round
  CosineROM : Constant  Value=fi(cos(deg2rad(theta)), 1, 16, 14)  VectorParams1D=off  OutDataTypeStr=fixdt(1,16,14)  SampleTime=-1
  CosineROM1 : Constant  Value=fi(sin(deg2rad(theta)), 1, 16, 14)  VectorParams1D=off  OutDataTypeStr=fixdt(1,16,14)  SampleTime=-1
  Selector : Selector  NumberOfDimensions=2  IndexMode=Zero-based  InputPortWidth=3  IndexOptions=Index vector (dialog),Index vector (port)  Indices=0,1  OutputSizes=1,1
  Selector1 : Selector  NumberOfDimensions=2  IndexMode=Zero-based  InputPortWidth=3  IndexOptions=Index vector (dialog),Index vector (port)  Indices=0,1  OutputSizes=1,1
  xcos : Product  OutDataTypeStr=fixdt(1, ceil(log2(w)), 0);  RndMeth=Round
  xcos1 : Product  OutDataTypeStr=fixdt(1, ceil(log2(h)), 0);  RndMeth=Round
  Rho : Outport  VectorParamsAs1DForOutWhenUnconnected=off
  wires:
  CosineROM/1 -> Selector/1
  Selector/1 -> xcos/2
  xcos/1 -> Add/1
  Add/1 -> Rho/1
  X/1 -> xcos/1
  Index/1 -> Selector/2, Selector1/2
  Selector1/1 -> xcos1/2
  xcos1/1 -> Add/2
  CosineROM1/1 -> Selector1/1
  Y/1 -> xcos1/1

== system hybrid_lht_accumulator_backup/Hybrid LHT2/Hybrid LHT Accumulator/Accumulator with Switches/Accumulator/Block RAM/Simple Dual Port RAM ==
  wr_data : Inport
  wr_addr : Inport  Port=2
  wr_en : Inport  Port=3
  rd_addr : Inport  Port=4
  Simple Dual Port RAM : hdlsllib/HDL RAMs/Simple Dual Port RAM  ram_size=ceil(log2(maxRho*2))
      settings: SourceProductName=Simulink  SourceProductBaseCode=SL
  rd_data : Outport
  wires:
  wr_data/1 -> Simple Dual Port RAM/1
  wr_addr/1 -> Simple Dual Port RAM/2
  wr_en/1 -> Simple Dual Port RAM/3
  rd_addr/1 -> Simple Dual Port RAM/4
  Simple Dual Port RAM/1 -> rd_data/1

== system hybrid_lht_accumulator_backup/Hybrid LHT2/Hybrid LHT Accumulator/Accumulator with Switches/Accumulator/Block RAM/Simple Dual Port RAM Generator ==
  wr_data : Inport
  wr_addr : Inport  Port=2
  wr_en : Inport  Port=3
  rd_addr : Inport  Port=4
  rd_address : hdlsllib/Logic and Bit Operations/Bit Slice  lidx=8  ridx=0
      settings: SourceProductName=Simulink  SourceProductBaseCode=SL
  simple_ram_0 : hdlsllib/HDL RAMs/Simple Dual Port RAM  ram_size=9
      settings: SourceProductName=Simulink  SourceProductBaseCode=SL
  wr_address : hdlsllib/Logic and Bit Operations/Bit Slice  lidx=8  ridx=0
      settings: SourceProductName=Simulink  SourceProductBaseCode=SL
  rd_data : Outport
  wires:
  wr_data/1 -> simple_ram_0/1
  wr_addr/1 -> wr_address/1
  wr_address/1 -> simple_ram_0/2
  wr_en/1 -> simple_ram_0/3
  rd_addr/1 -> rd_address/1
  rd_address/1 -> simple_ram_0/4
  simple_ram_0/1 -> rd_data/1

== matlab function hybrid_lht_accumulator_backup/Hybrid LHT2/Hybrid LHT Accumulator/Accumulator Controller ==
  data: shift output; sof input; mode output; eof input; read output; clear output; index output; ntheta input; nrho input; valid output; nshift input
function [shift, mode, read, clear, index, valid] = fcn(sof, eof, ntheta, nrho, nshift)

IDLE = fi(0, 0, 2, 0);
VOTE = fi(1, 0, 2, 0);
READ = fi(2, 0, 2, 0);
CLEAR = fi(3, 0, 2, 0);

persistent current_state;
persistent rho_counter;
persistent theta_counter;
persistent shift_counter;

if isempty(current_state)
    current_state = IDLE;
end

if isempty(rho_counter)
    rho_counter = fi(0, 0, 16, 0);
end

if isempty(theta_counter)
    theta_counter = fi(0, 0, 16, 0);
end

if isempty(shift_counter)
    shift_counter = fi(0, 0, 16, 0);
end

switch current_state
    case IDLE
        rho_counter = fi(0, 0, 16, 0);
        theta_counter = fi(0, 0, 16, 0);
        shift_counter = fi(0, 0, 16, 0);
        
        clear = false;
        valid = false;
        
        read = rho_counter;
        index = theta_counter;
        shift = shift_counter;
        
        if sof
            mode = true;
            current_state = VOTE;
        else
            mode = false;
            current_state = IDLE;
        end
        
    case VOTE
        rho_counter = fi(0, 0, 16, 0);
        theta_counter = fi(0, 0, 16, 0);
        shift_counter = fi(0, 0, 16, 0);
        
        mode = true;
        clear = false;
        valid = false;
        
        shift = shift_counter;
        read = rho_counter;
        index = theta_counter;
        
        if eof
            current_state = READ;
        else
            current_state = VOTE;
        end
        
    case READ
        mode = false;
        clear = false;
        valid = true;
        
        read = rho_counter;
        index = theta_counter;
        shift = shift_counter;
        
        if theta_counter >= ntheta && rho_counter >= nrho && shift_counter >= nshift
            rho_counter = fi(0, 0, 16, 0);
            theta_counter = fi(0, 0, 16, 0);
            shift_counter = fi(0, 0, 16, 0);
            current_state = CLEAR;
        elseif theta_counter >= ntheta && rho_counter >= nrho
            theta_counter = fi(0, 0, 16, 0);
            rho_counter = fi(0, 0, 16, 0);
            shift_counter = fi(shift_counter + 1, 0, 16, 0);
            current_state = READ;
        elseif rho_counter >= nrho
            rho_counter = fi(0, 0, 16, 0);
            theta_counter = fi(theta_counter + 1, 0, 16, 0);
            current_state = READ;
        else
            rho_counter = fi(rho_counter + 1, 0, 16, 0);
            current_state = READ;
        end
        
    case CLEAR
        mode = false;
        clear = true;
        valid = false;
        
        read = rho_counter;
        index = theta_counter;
        shift = shift_counter;
        
        if rho_counter >= nrho
            rho_counter = fi(0, 0, 16, 0);
            theta_counter = fi(0, 0, 16, 0);
            shift_counter = fi(0, 0, 16, 0);
            current_state = IDLE;
        else
            rho_counter = fi(rho_counter + 1, 0, 16, 0);
            theta_counter = fi(0, 0, 16, 0);
            shift_counter = fi(0, 0, 16, 0);
            current_state = CLEAR;
        end
        
    otherwise
        rho_counter = fi(0, 0, 16, 0);
        theta_counter = fi(0, 0, 16, 0);
        shift_counter = fi(0, 0, 16, 0);
        
        mode = false;
        clear = false;
        valid = false;
        
        shift = shift_counter;
        read = rho_counter;
        index = theta_counter;
        
        current_state = IDLE;
        
end

== matlab function hybrid_lht_accumulator_backup/Hybrid LHT2/Hybrid LHT Accumulator2/Accumulator Control ==
  data: shift output; clear output; address output; sel output; read output; idx output; sof input; eof input; fvalid input; hStart output; hEnd output; vStart output; vEnd output; valid output; mode input; ready input; rhomax input; thetamax input; debug_state output; shiftmax input
function [shift, clear, address, sel, read, idx, hStart, hEnd, vStart, vEnd, valid, debug_state]  = acc_fsm(sof, eof, fvalid, mode, ready, rhomax, thetamax, shiftmax)

IDLE = fi(0, 0, 3, 0);
VOTE = fi(1, 0, 3, 0);
BACKPROP = fi(2, 0, 3, 0);
READ = fi(3, 0, 3, 0);
CLEAR = fi(7, 0 , 3, 0);

persistent rhocounter;

persistent thetacounter;

persistent shiftcounter;

persistent current_state;

if isempty(rhocounter)
    rhocounter = fi(0, 0, 32, 0);
end

if isempty(thetacounter)
    thetacounter = fi(0, 0, 32, 0);
end

if isempty(shiftcounter)
    shiftcounter = fi(0, 0, 6, 0);
end

if isempty(current_state)
    current_state = IDLE;
end

switch current_state
    case IDLE
        % Set Control Output
        clear = false;
        address = rhocounter;
        read = false;
        idx = thetacounter;
        shift = shiftcounter;
        
        % Set debug
        debug_state = current_state;
        
        % Set Video Output
        hStart = false;
        hEnd = false;
        vStart = false;
        vEnd = false;
        valid = false;
        
        % Set Variables
        rhocounter = fi(0, 0, 32, 0);
        thetacounter = fi(0, 0, 32, 0);
        shiftcounter = fi(0, 0, 6, 0);
        
        % Set next state
        if sof && fvalid
            sel = true;
            current_state = VOTE;
        else
            sel = false;
            current_state = IDLE;
        end
        
    case VOTE
        % Set Control Output
        clear = false;
        address = rhocounter;
        sel = true;
        read = false;
        idx = thetacounter;
        shift = shiftcounter;
        
        % Set debug
        debug_state = current_state;
        
        % Set Video Output
        hStart = false;
        hEnd = false;
        vStart = false;
        vEnd = false;
        valid = false;
        
        % Set Variables
        rhocounter = fi(0, 0, 32, 0);
        thetacounter = fi(0, 0, 32, 0);
        shiftcounter = fi(0, 0, 6, 0);
        
        % Set next state
        if eof && fvalid
            if mode
                current_state = BACKPROP;
            else
                current_state = READ;
            end
        else
            current_state = VOTE;
        end
         
    case BACKPROP
        % Set Control Output
        clear = true;
        address = rhocounter;
        sel = false;
        read = true;
        idx = thetacounter;
        shift = shiftcounter;
        
        % Set debug
        debug_state = current_state;
        
        shiftcounter = fi(0, 0, 6, 0);
        
        % Set Video Output
        hStart = false;
        hEnd = false;
        vStart = false;
        vEnd = false;
        valid = false;
        
        % Set next state
        if rhocounter >= rhomax
            current_state = IDLE;
        else
            % Set Variables
            rhocounter = fi(rhocounter + 1, 0, 32, 0);
            thetacounter = fi(0, 0, 32, 0);
            current_state = BACKPROP;
        end
        
    case READ
        % Set Control Output
        clear = false;
        address = rhocounter;
        sel = false;
        read = false;
        idx = thetacounter;
        shift = shiftcounter;
        
        % Set debug
        debug_state = current_state;
        
        % Set Video Output
        if rhocounter == 0
            hStart = true;
        else
            hStart = false;
        end
        
        if rhocounter == rhomax
            hEnd = true;
        else
            hEnd = false;
        end
        
        if rhocounter == 0 && thetacounter == 0 && shiftcounter == 0
            vStart = true;
        else
            vStart = false;
        end
        
        if rhocounter == rhomax && thetacounter == thetamax && shiftcounter == shiftmax
            vEnd = true;
        else
            vEnd = false;
        end
        
        if ready
            valid = true;
        else
            valid = false;
        end
        
        % Set next state
        if rhocounter >= rhomax && thetacounter >= thetamax && shiftcounter >= shiftmax
            rhocounter = fi(0, 0, 32, 0);
            thetacounter = fi(0, 0, 32, 0);
            shiftcounter = fi(0, 0, 6, 0);
            current_state = CLEAR;
        else
            if ready
                % Set Variables
                if thetacounter >= thetamax && rhocounter >= rhomax
                    rhocounter = fi(0, 0, 32, 0);
                    thetacounter = fi(0, 0, 32, 0);
                    shiftcounter = fi(shiftcounter + 1, 0, 6, 0);

                elseif rhocounter >= rhomax
                    rhocounter = fi(0, 0, 32, 0);
                    thetacounter = fi(thetacounter + 1, 0, 32, 0);

                else
                    rhocounter = fi(rhocounter + 1, 0, 32, 0);
                end
            end

            current_state = READ;
        end
        
    case CLEAR
        % Set Control Output
        clear = true;
        address = rhocounter;
        sel = false;
        read = false;
        idx = thetacounter;
        shift = shiftcounter;
        
        % Set debug
        debug_state = current_state;
        
        % Set Video Output
        hStart = false;
        hEnd = false;
        vStart = false;
        vEnd = false;
        valid = false;

        % Set next state
        if rhocounter >= rhomax
            current_state = IDLE;
        else
            % Set Variables
            rhocounter = fi(rhocounter + 1, 0, 32, 0);
            thetacounter = fi(0, 0, 32, 0);
            current_state = CLEAR;
        end
        
    otherwise
        % Set Control Output
        clear = false;
        address = rhocounter;
        sel = true;
        read = false;
        idx = thetacounter;
        shift = shiftcounter;
        
        % Set debug
        debug_state = current_state;
        
        % Set Video Output
        hStart = false;
        hEnd = false;
        vStart = false;
        vEnd = false;
        valid = false;
        
        % Set Variables
        rhocounter = fi(0, 0, 32, 0);
        thetacounter = fi(0, 0, 32, 0);
        
        % Set next state
        current_state = IDLE;
        
end
end
